simulink model "CSE_BDA__SIMULINK_NO1_DIPASUPIL_MAGSINO"  (R2019a)
settings: Solver=VariableStepAuto  StartTime=0.0  StopTime=20  RelTol=1e-3
undefined symbols (not defined in the file): G1_den, G1_num, G2_den, G2_num, G3_den, G3_num, H1_den, H1_num, H2_den, H2_num, H3_den, H3_num, T_F2den, T_F2num, TF_G1G2H2_den, TF_G1G2H2_num, TF_G1G2H2H1_den, TF_G1G2H2H1_num, TF_G3H3recipG2_den, TF_G3H3recipG2_num, TF_reduced_den, TF_reduced_num
settings Model: Creator=User  LastModifiedBy=User

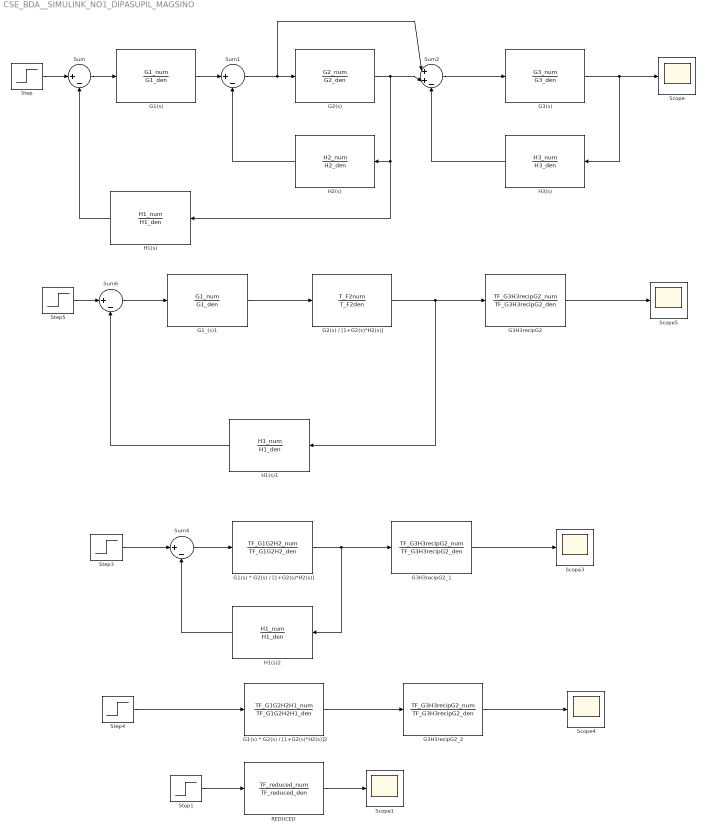
== system CSE_BDA__SIMULINK_NO1_DIPASUPIL_MAGSINO ==
  G1(s) : TransferFcn  Numerator=G1_num  Denominator=G1_den
  G1(s) * G2(s) / [1+G2(s)*H2(s)] : TransferFcn  Numerator=TF_G1G2H2_num  Denominator=TF_G1G2H2_den
  G1(s) * G2(s) / [1+G2(s)*H2(s)]2 : TransferFcn  Numerator=TF_G1G2H2H1_num  Denominator=TF_G1G2H2H1_den
  G1_(s)1 : TransferFcn  Numerator=G1_num  Denominator=G1_den
  G2(s) : TransferFcn  Numerator=G2_num  Denominator=G2_den
  G2(s) / [1+G2(s)*H2(s)] : TransferFcn  Numerator=T_F2num  Denominator=T_F2den
  G3(s) : TransferFcn  Numerator=G3_num  Denominator=G3_den
  G3H3recipG2 : TransferFcn  Numerator=TF_G3H3recipG2_num  Denominator=TF_G3H3recipG2_den
  G3H3recipG2_1 : TransferFcn  Numerator=TF_G3H3recipG2_num  Denominator=TF_G3H3recipG2_den
  G3H3recipG2_2 : TransferFcn  Numerator=TF_G3H3recipG2_num  Denominator=TF_G3H3recipG2_den
  H1(s) : TransferFcn  Numerator=H1_num  Denominator=H1_den
  H1(s)1 : TransferFcn  Numerator=H1_num  Denominator=H1_den
  H1(s)2 : TransferFcn  Numerator=H1_num  Denominator=H1_den
  H2(s) : TransferFcn  Numerator=H2_num  Denominator=H2_den
  H3(s) : TransferFcn  Numerator=H3_num  Denominator=H3_den
  REDUCED : TransferFcn  Numerator=TF_reduced_num  Denominator=TF_reduced_den
  Scope{,1,3..5} (5 alike) : Scope
  Step{,1,3..5} (5 alike) : Step  SampleTime=0
  Sum{,1,4,6} (4 alike) : Sum  Inputs=|+-
  Sum2 : Sum  Inputs=|++-
  wires:
  Step/1 -> Sum/1
  Sum/1 -> G1(s)/1
  G1(s)/1 -> Sum1/1
  H1(s)/1 -> Sum/2
  Sum1/1 -> Sum2/1, G2(s)/1
  G2(s)/1 -> H1(s)/1, H2(s)/1, Sum2/2
  Sum2/1 -> G3(s)/1
  G3(s)/1 -> H3(s)/1, Scope/1
  H2(s)/1 -> Sum1/2
  H3(s)/1 -> Sum2/3
  Step1/1 -> REDUCED/1
  REDUCED/1 -> Scope1/1
  Step3/1 -> Sum4/1
  H1(s)2/1 -> Sum4/2
  Sum4/1 -> G1(s) * G2(s) / [1+G2(s)*H2(s)]/1
  G1(s) * G2(s) / [1+G2(s)*H2(s)]/1 -> H1(s)2/1, G3H3recipG2_1/1
  G3H3recipG2/1 -> Scope5/1
  G2(s) / [1+G2(s)*H2(s)]/1 -> G3H3recipG2/1, H1(s)1/1
  G1_(s)1/1 -> G2(s) / [1+G2(s)*H2(s)]/1
  Step5/1 -> Sum6/1
  H1(s)1/1 -> Sum6/2
  Sum6/1 -> G1_(s)1/1
  G3H3recipG2_1/1 -> Scope3/1
  G1(s) * G2(s) / [1+G2(s)*H2(s)]2/1 -> G3H3recipG2_2/1
  G3H3recipG2_2/1 -> Scope4/1
  Step4/1 -> G1(s) * G2(s) / [1+G2(s)*H2(s)]2/1
